simulink model "Lab2_simulation"  (R2023a)
settings: Solver=ode45  StartTime=0.0  StopTime=10.0  RelTol=1e-3
settings Model: Creator=amylang2  LastModifiedBy=amylang2

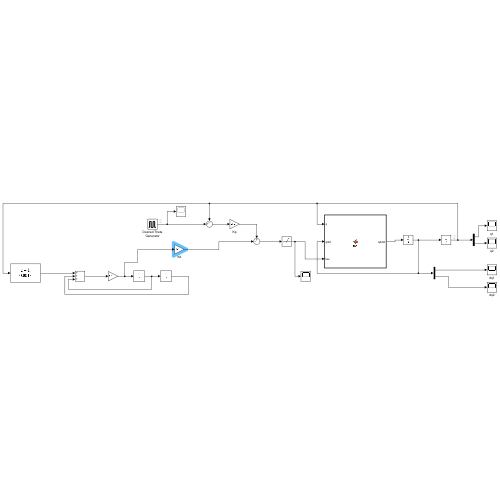
[thumbnail: Simulink's stored preview of the top-level diagram]
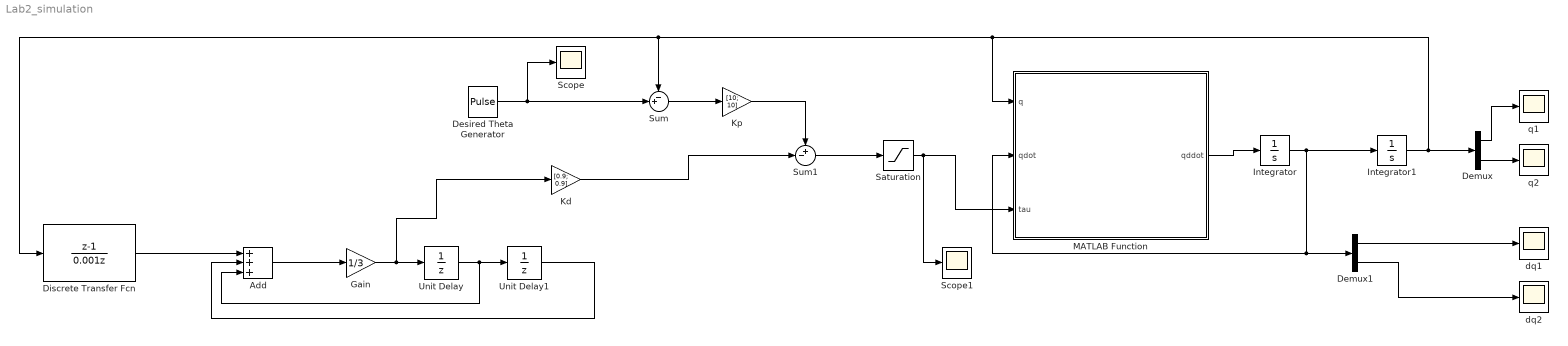
== system Lab2_simulation ==
  Add : Sum  Inputs=+++
  Demux : Demux  Outputs=2
  Demux1 : Demux  Outputs=2
  Desired Theta Generator : DiscretePulseGenerator  PulseType=Time based  Amplitude=pi/6  PulseWidth=50
  Discrete Transfer Fcn : DiscreteTransferFcn  Numerator=[1 -1]  Denominator=[0.001 0]  SampleTime=.001
  Gain : Gain  Gain=1/3
  Integrator : Integrator
  Integrator1 : Integrator  InitialCondition=[0;0]
  Kd : Gain  Gain=[0.9; 0.9]
  Kp : Gain  Gain=[10; 10]
  MATLAB Function : MATLAB Function  TreatAsAtomicUnit=on
  Saturation : Saturate  UpperLimit=5  LowerLimit=-5
  Scope : Scope
  Scope1 : Scope
  Sum : Sum  Inputs=-+|
  Sum1 : Sum  Inputs=+-|
  Unit Delay : UnitDelay  SampleTime=0.001  HasFrameUpgradeWarning=on
  Unit Delay1 : UnitDelay  SampleTime=.001  HasFrameUpgradeWarning=on
  dq1 : Scope
  dq2 : Scope
  q1 : Scope
  q2 : Scope
  wires:
  Sum1/1 -> Saturation/1
  Integrator/1 -> Integrator1/1, MATLAB Function/2(qdot), Demux1/1
  MATLAB Function/1(qddot) -> Integrator/1
  Demux/1 -> q1/1
  Demux/2 -> q2/1
  Demux1/1 -> dq1/1
  Demux1/2 -> dq2/1
  Integrator1/1 -> Discrete Transfer Fcn/1, Sum/1, MATLAB Function/1(q), Demux/1
  Discrete Transfer Fcn/1 -> Add/1
  Add/1 -> Gain/1
  Gain/1 -> Kd/1, Unit Delay/1
  Unit Delay/1 -> Add/3, Unit Delay1/1
  Unit Delay1/1 -> Add/2
  Desired Theta Generator/1 -> Scope/1, Sum/2
  Sum/1 -> Kp/1
  Kp/1 -> Sum1/1
  Kd/1 -> Sum1/2
  Saturation/1 -> Scope1/1, MATLAB Function/3(tau)

== matlab function Lab2_simulation/MATLAB Function ==
  data: q input; qddot output; qdot input; tau input
function qddot = fcn(q, qdot, tau)
qddot = [0;0];

theta2 = q(1);
theta3 = q(2);

omega2 = qdot(1);
omega3 = qdot(2);

p1 = 0.03;
p2 = 0.0128;
p3 = 0.0076;
p4 = 0.0753;
p5 = 0.0298;

% gravity acceleration constant
g = 9.81;

D = [p1 -p3*sin(theta3-theta2); -p3*sin(theta3 - theta2) p2];
C = [0 -p3*cos(theta3 - theta2)*omega3; p3*cos(theta3 - theta2)*omega2 0];
G = [-p4*g*sin(theta2); -p5*g*cos(theta3)];

qddot = inv(D)*tau - inv(D)*C*qdot - inv(D)*G;
end
